simulink model "SIMULINK_FT_SRL_NZS_Tracking_R18b"  (R2018b)
settings: Solver=FixedStepAuto  StartTime=0.0  StopTime=sim_end_time  FixedStep=fixed_step_size  RelTol=1e-3
InitFcn:
  | start_uav_car_10
values from neighbouring files (symbols this model uses):
  a = 1    [start_uav_car_10.m]
  act_end = 2*pi/w1    (= 62.8318530718)    [start_uav_car_10.m]
  b = 1.8    [start_uav_car_10.m]
  battery_threshold = 20    [start_uav_car_10.m]
  bb = 1.2    [start_uav_car_10.m]
  delta_ = [delta_his(2:end,:); delta]    [adp_tracking.m]    (also in start_uav_car_10.m = zeros(N,1))
  draw_gif = false    [start_uav_car_10.m]
  fixed_step_size = 1/30    (= 0.0333333333333)    [start_uav_car_10.m]
  k = 0.2    [start_uav_car_10.m]
  KD_x = 0.000002    (= 2e-06)    [start_uav_car_10.m]
  KD_y = 0.00002    (= 2e-05)    [start_uav_car_10.m]
  kd_z = 0.02    [start_uav_car_10.m]
  KDD_x = 0.0008    [start_uav_car_10.m]
  KDD_y = 0.0008    [start_uav_car_10.m]
  KI_x = 0.000002    (= 2e-06)    [start_uav_car_10.m]
  KI_y = 0.000002    (= 2e-06)    [start_uav_car_10.m]
  ki_z = 0.002    [start_uav_car_10.m]
  KII_x = 0.000000    (= 0)    [start_uav_car_10.m]
  KII_y = 0.000    (= 0)    [start_uav_car_10.m]
  KP_x = 1.5    [start_uav_car_10.m]
  KP_y = 1.5    [start_uav_car_10.m]
  kp_z = 0.7    [start_uav_car_10.m]
  KPP_x = 0.4    [start_uav_car_10.m]
  KPP_y = 0.4    [start_uav_car_10.m]
  lmt = 0.5    [start_uav_car_10.m]
  omega = omega_(i,:)    [adp_tracking.m]    (also in start_uav_car_10.m = 0.3)
  omega_ = [omega_his(2:end,:); omega']    [adp_tracking.m]    (also in start_uav_car_10.m = zeros(N,l))
  R = 200*eye(2)    [adp_tracking.m]    (also in start_uav_car_10.m = 0.7)
  sim_end_time = 300    [start_uav_car_10.m]    (also in trjcar.m = 600)
  UAV_NUM = 1    [start_uav_car_10.m]
  Vel_Switch_1 = 1    [start_uav_car_10.m]
  Vel_Switch_10 = 1    [start_uav_car_10.m]
  Vel_Switch_11 = 1    [start_uav_car_10.m]
  Vel_Switch_12 = 1    [start_uav_car_10.m]
  Vel_Switch_13 = 1    [start_uav_car_10.m]
  Vel_Switch_14 = 1    [start_uav_car_10.m]
  Vel_Switch_15 = 1    [start_uav_car_10.m]
  Vel_Switch_16 = 1    [start_uav_car_10.m]
  Vel_Switch_17 = 1    [start_uav_car_10.m]
  Vel_Switch_18 = 1    [start_uav_car_10.m]
  Vel_Switch_19 = 1    [start_uav_car_10.m]
  Vel_Switch_2 = 1    [start_uav_car_10.m]
  Vel_Switch_20 = 1    [start_uav_car_10.m]
  Vel_Switch_3 = 1    [start_uav_car_10.m]
  Vel_Switch_4 = 1    [start_uav_car_10.m]
  Vel_Switch_5 = 1    [start_uav_car_10.m]
  Vel_Switch_6 = 1    [start_uav_car_10.m]
  Vel_Switch_7 = 1    [start_uav_car_10.m]
  Vel_Switch_8 = 1    [start_uav_car_10.m]
  Vel_Switch_9 = 1    [start_uav_car_10.m]
  W0 = 10*ones(l,1)    [start_uav_car_10.m]
  w1 = 0.1    [start_uav_car_10.m]
  w2 = 30    [start_uav_car_10.m]
  XMAX = 2.8    [start_uav_car_10.m]
  XMIN = -2.8    [start_uav_car_10.m]
  YMAX = 2.2    [start_uav_car_10.m]
  YMIN = -2.2    [start_uav_car_10.m]
  ys = ys_learned - ys_learned(1,:)    [start_uav_car_10.m]
  ys_learned = [-20 -19.9842645881 -19.9722755737 -19.9635643089 -19.9577075469 -19.9543235714 -19.9530686431 -19.9536337356 -19.9557415391 -19.9591437091 -19.9636183405 -19.9689676484 ... (12618 elements, 6309x2)]    [DMP_ref.mat]
  z_d_for_land = 1    [start_uav_car_10.m]
  ZMAX = 2.0    (= 2)    [start_uav_car_10.m]
  ZMIN = 0.7    [start_uav_car_10.m]
undefined symbols (not defined in the file or in its folder): droneyeeUAV2_NUM, droneyeeUAV3_NUM, droneyeeUAV4_NUM, droneyeeUAV5_NUM, uav10num, uav1num, uav2num, uav3num, uav4num, uav5num, uav6num, uav7num, uav8num, uav9num
libraries: simulink x121, aerolibanimutils x1
(part 9 of 11)

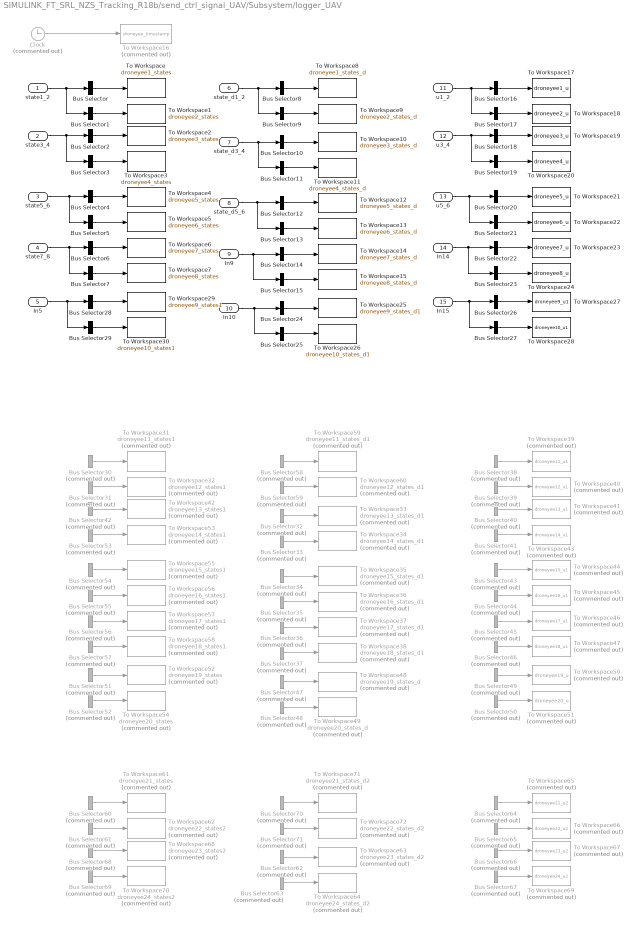
== system SIMULINK_FT_SRL_NZS_Tracking_R18b/send_ctrl_signal_UAV/Subsystem/logger_UAV ==
  state1_2 : Inport
  state3_4 : Inport  Port=2
  state5_6 : Inport  Port=3
  state7_8 : Inport  Port=4
  In5 : Inport  Port=5
  state_d1_2 : Inport  Port=6
  state_d3_4 : Inport  Port=7
  state_d5_6 : Inport  Port=8
  In9 : Inport  Port=9
  In10 : Inport  Port=10
  u1_2 : Inport  Port=11
  u3_4 : Inport  Port=12
  u5_6 : Inport  Port=13
  In14 : Inport  Port=14
  In15 : Inport  Port=15
  Bus Selector : BusSelector  OutputSignals=droneyeeUAV1_states.x,droneyeeUAV1_states.y,droneyeeUAV1_states.z,droneyeeUAV1_states.roll,droneyeeUAV1_states.pitch,droneyeeUAV1_states.yaw  OutputAsBus=on
  Bus Selector1 : BusSelector  OutputSignals=droneyeeUAV2_states.x,droneyeeUAV2_states.y,droneyeeUAV2_states.z,droneyeeUAV2_states.roll,droneyeeUAV2_states.pitch,droneyeeUAV2_states.yaw  OutputAsBus=on
  Bus Selector10 : BusSelector  OutputSignals=droneyeeUAV3_d.x3_d,droneyeeUAV3_d.y3_d,droneyeeUAV3_d.z3_d,droneyeeUAV3_d.yaw3_d  OutputAsBus=on
  Bus Selector11 : BusSelector  OutputSignals=droneyeeUAV4_d.x4_d,droneyeeUAV4_d.y4_d,droneyeeUAV4_d.z4_d,droneyeeUAV4_d.yaw4_d  OutputAsBus=on
  Bus Selector12 : BusSelector  OutputSignals=droneyeeUAV5_d.x5_d,droneyeeUAV5_d.y5_d,droneyeeUAV5_d.z5_d,droneyeeUAV5_d.yaw5_d  OutputAsBus=on
  Bus Selector13 : BusSelector  OutputSignals=droneyeeUAV6_d  OutputAsBus=on
  Bus Selector14 : BusSelector  OutputSignals=droneyeeUAV7_d  OutputAsBus=on
  Bus Selector15 : BusSelector  OutputSignals=droneyeeUAV8_d  OutputAsBus=on
  Bus Selector16 : BusSelector  OutputSignals=uav1.u_vx,uav1.u_vy,uav1.u_vz,uav1.u_rate_roll,uav1.u_rate_pitch,uav1.u_rate_yaw  OutputAsBus=on
  Bus Selector17 : BusSelector  OutputSignals=uav2.u_vx,uav2.u_vy,uav2.u_vz,uav2.u_rate_roll,uav2.u_rate_pitch,uav2.u_rate_yaw  OutputAsBus=on
  Bus Selector18 : BusSelector  OutputSignals=uav3.u_vx,uav3.u_vy,uav3.u_vz,uav3.u_rate_roll,uav3.u_rate_pitch,uav3.u_rate_yaw  OutputAsBus=on
  Bus Selector19 : BusSelector  OutputSignals=uav4.u_vx,uav4.u_vy,uav4.u_vz,uav4.u_rate_roll,uav4.u_rate_pitch,uav4.u_rate_yaw  OutputAsBus=on
  Bus Selector2 : BusSelector  OutputSignals=droneyeeUAV3_states.x,droneyeeUAV3_states.y,droneyeeUAV3_states.z,droneyeeUAV3_states.roll,droneyeeUAV3_states.pitch,droneyeeUAV3_states.yaw  OutputAsBus=on
  Bus Selector20 : BusSelector  OutputSignals=uav_5.u_vx,uav_5.u_vy,uav_5.u_vz,uav_5.u_rate_roll,uav_5.u_rate_pitch,uav_5.u_rate_yaw  OutputAsBus=on
  Bus Selector21 : BusSelector  OutputSignals=uav_6  OutputAsBus=on
  Bus Selector22 : BusSelector  OutputSignals=uav_7  OutputAsBus=on
  Bus Selector23 : BusSelector  OutputSignals=uav_8  OutputAsBus=on
  Bus Selector24 : BusSelector  OutputSignals=droneyeeUAV9_d  OutputAsBus=on
  Bus Selector25 : BusSelector  OutputSignals=droneyeeUAV10_d  OutputAsBus=on
  Bus Selector26 : BusSelector  OutputSignals=uav_9  OutputAsBus=on
  Bus Selector27 : BusSelector  OutputSignals=uav_10  OutputAsBus=on
  Bus Selector28 : BusSelector  OutputSignals=droneyeeUAV9_states  OutputAsBus=on
  Bus Selector29 : BusSelector  OutputSignals=droneyeeUAV10_states  OutputAsBus=on
  Bus Selector3 : BusSelector  OutputSignals=droneyeeUAV4_states.x,droneyeeUAV4_states.y,droneyeeUAV4_states.z,droneyeeUAV4_states.roll,droneyeeUAV4_states.pitch,droneyeeUAV4_states.yaw  OutputAsBus=on
  Bus Selector30 : BusSelector  Commented=on  OutputSignals=droneyeeUAV11_states.x1,droneyeeUAV11_states.y1,droneyeeUAV11_states.z1,droneyeeUAV11_states.yaw1,droneyeeUAV11_states.vx1,droneyeeUAV11_states.vy1,droneyeeUAV11_states.vz1  OutputAsBus=on
  Bus Selector31 : BusSelector  Commented=on  OutputSignals=droneyeeUAV12_states.x2,droneyeeUAV12_states.y2,droneyeeUAV12_states.z2,droneyeeUAV12_states.yaw2,droneyeeUAV12_states.vx2,droneyeeUAV12_states.vy2,droneyeeUAV12_states.vz2  OutputAsBus=on
  Bus Selector32 : BusSelector  Commented=on  OutputSignals=droneyeeUAV13_d.x13_d,droneyeeUAV13_d.y13_d,droneyeeUAV13_d.z13_d,droneyeeUAV13_d.yaw13_d  OutputAsBus=on
  Bus Selector33 : BusSelector  Commented=on  OutputSignals=droneyeeUAV14_d.x14_d,droneyeeUAV14_d.y14_d,droneyeeUAV14_d.z14_d,droneyeeUAV14_d.yaw14_d  OutputAsBus=on
  Bus Selector34 : BusSelector  Commented=on  OutputSignals=droneyeeUAV15_d.x15_d,droneyeeUAV15_d.y15_d,droneyeeUAV15_d.z15_d,droneyeeUAV15_d.yaw15_d  OutputAsBus=on
  Bus Selector35 : BusSelector  Commented=on  OutputSignals=droneyeeUAV16_d.x16_d,droneyeeUAV16_d.y16_d,droneyeeUAV16_d.z16_d,droneyeeUAV16_d.yaw16_d  OutputAsBus=on
  Bus Selector36 : BusSelector  Commented=on  OutputSignals=droneyeeUAV17_d.x17_d,droneyeeUAV17_d.y17_d,droneyeeUAV17_d.z17_d,droneyeeUAV17_d.yaw17_d  OutputAsBus=on
  Bus Selector37 : BusSelector  Commented=on  OutputSignals=droneyeeUAV18_d.x18_d,droneyeeUAV18_d.y18_d,droneyeeUAV18_d.z18_d,droneyeeUAV18_d.yaw18_d  OutputAsBus=on
  Bus Selector38 : BusSelector  Commented=on  OutputSignals=uav1.u_vx,uav1.u_vy,uav1.u_vz,uav1.u_rate_roll,uav1.u_rate_pitch,uav1.u_rate_yaw  OutputAsBus=on
  Bus Selector39 : BusSelector  Commented=on  OutputSignals=uav2.u_vx,uav2.u_vy,uav2.u_vz,uav2.u_rate_roll,uav2.u_rate_pitch,uav2.u_rate_yaw  OutputAsBus=on
  Bus Selector4 : BusSelector  OutputSignals=droneyeeUAV5_states.x,droneyeeUAV5_states.y,droneyeeUAV5_states.z,droneyeeUAV5_states.roll,droneyeeUAV5_states.pitch,droneyeeUAV5_states.yaw  OutputAsBus=on
  Bus Selector40 : BusSelector  Commented=on  OutputSignals=uav3.u_vx,uav3.u_vy,uav3.u_vz,uav3.u_rate_roll,uav3.u_rate_pitch,uav3.u_rate_yaw  OutputAsBus=on
  Bus Selector41 : BusSelector  Commented=on  OutputSignals=uav4.u_vx,uav4.u_vy,uav4.u_vz,uav4.u_rate_roll,uav4.u_rate_pitch,uav4.u_rate_yaw  OutputAsBus=on
  Bus Selector42 : BusSelector  Commented=on  OutputSignals=droneyeeUAV13_states.x3,droneyeeUAV13_states.y3,droneyeeUAV13_states.z3,droneyeeUAV13_states.yaw3,droneyeeUAV13_states.vx3,droneyeeUAV13_states.vy3,droneyeeUAV13_states.vz3  OutputAsBus=on
  Bus Selector43 : BusSelector  Commented=on  OutputSignals=uav5.u_vx,uav5.u_vy,uav5.u_vz,uav5.u_rate_roll,uav5.u_rate_pitch,uav5.u_rate_yaw  OutputAsBus=on
  Bus Selector44 : BusSelector  Commented=on  OutputSignals=uav6.u_vx,uav6.u_vy,uav6.u_vz,uav6.u_rate_roll,uav6.u_rate_pitch,uav6.u_rate_yaw  OutputAsBus=on
  Bus Selector45 : BusSelector  Commented=on  OutputSignals=uav7.u_vx,uav7.u_vy,uav7.u_vz,uav7.u_rate_roll,uav7.u_rate_pitch,uav7.u_rate_yaw  OutputAsBus=on
  Bus Selector46 : BusSelector  Commented=on  OutputSignals=uav8.u_vx,uav8.u_vy,uav8.u_vz,uav8.u_rate_roll,uav8.u_rate_pitch,uav8.u_rate_yaw  OutputAsBus=on
  Bus Selector47 : BusSelector  Commented=on  OutputSignals=droneyeeUAV19_d.x19_d,droneyeeUAV19_d.y19_d,droneyeeUAV19_d.z19_d,droneyeeUAV19_d.yaw19_d  OutputAsBus=on
  Bus Selector48 : BusSelector  Commented=on  OutputSignals=droneyeeUAV20_d.x20_d,droneyeeUAV20_d.y20_d,droneyeeUAV20_d.z20_d,droneyeeUAV20_d.yaw20_d  OutputAsBus=on
  Bus Selector49 : BusSelector  Commented=on  OutputSignals=uav9.u_vx,uav9.u_vy,uav9.u_vz,uav9.u_rate_roll,uav9.u_rate_pitch,uav9.u_rate_yaw  OutputAsBus=on
  Bus Selector5 : BusSelector  OutputSignals="droneyeeUAV6_states.x,droneyeeUAV6_states.y,droneyeeUAV6_states.z,droneyeeUAV6_states.roll,droneyeeUAV6_states.pitch,droneyeeUAV6_states.yaw,droneyeeUAV6_states.latitude(degE7),droneyeeUAV6_states.longitude\t(degE7),droneyeeUAV6_states.alttude(mm),droneyeeUAV6_states.x(home position),droneyeeUAV6_states.y(home position),droneyeeUAV6_states.z(home position)"  OutputAsBus=on
  Bus Selector50 : BusSelector  Commented=on  OutputSignals=uav10.u_vx,uav10.u_vy,uav10.u_vz,uav10.u_rate_roll,uav10.u_rate_pitch,uav10.u_rate_yaw  OutputAsBus=on
  Bus Selector51 : BusSelector  Commented=on  OutputSignals=droneyeeUAV19_states.x9,droneyeeUAV19_states.y9,droneyeeUAV19_states.z9,droneyeeUAV19_states.yaw9,droneyeeUAV19_states.vx9,droneyeeUAV19_states.vy9,droneyeeUAV19_states.vz9  OutputAsBus=on
  Bus Selector52 : BusSelector  Commented=on  OutputSignals=droneyeeUAV20_states.x10,droneyeeUAV20_states.y10,droneyeeUAV20_states.z10,droneyeeUAV20_states.yaw10,droneyeeUAV20_states.vx10,droneyeeUAV20_states.vy10,droneyeeUAV20_states.vz10  OutputAsBus=on
  Bus Selector53 : BusSelector  Commented=on  OutputSignals=droneyeeUAV14_states.x4,droneyeeUAV14_states.y4,droneyeeUAV14_states.z4,droneyeeUAV14_states.yaw4,droneyeeUAV14_states.vx4,droneyeeUAV14_states.vy4,droneyeeUAV14_states.vz4  OutputAsBus=on
  Bus Selector54 : BusSelector  Commented=on  OutputSignals=droneyeeUAV15_states.x5,droneyeeUAV15_states.y5,droneyeeUAV15_states.z5,droneyeeUAV15_states.yaw5,droneyeeUAV15_states.vx5,droneyeeUAV15_states.vy5,droneyeeUAV15_states.vz5  OutputAsBus=on
  Bus Selector55 : BusSelector  Commented=on  OutputSignals=droneyeeUAV16_states.x6,droneyeeUAV16_states.y6,droneyeeUAV16_states.z6,droneyeeUAV16_states.yaw6,droneyeeUAV16_states.vx6,droneyeeUAV16_states.vy6,droneyeeUAV16_states.vz6  OutputAsBus=on
  Bus Selector56 : BusSelector  Commented=on  OutputSignals=droneyeeUAV17_states.x7,droneyeeUAV17_states.y7,droneyeeUAV17_states.z7,droneyeeUAV17_states.yaw7,droneyeeUAV17_states.vx7,droneyeeUAV17_states.vy7,droneyeeUAV17_states.vz7  OutputAsBus=on
  Bus Selector57 : BusSelector  Commented=on  OutputSignals=droneyeeUAV18_states.x8,droneyeeUAV18_states.y8,droneyeeUAV18_states.z8,droneyeeUAV18_states.yaw8,droneyeeUAV18_states.vx8,droneyeeUAV18_states.vy8,droneyeeUAV18_states.vz8  OutputAsBus=on
  Bus Selector58 : BusSelector  Commented=on  OutputSignals=droneyeeUAV11_d.x11_d,droneyeeUAV11_d.y11_d,droneyeeUAV11_d.z11_d,droneyeeUAV11_d.yaw11_d  OutputAsBus=on
  Bus Selector59 : BusSelector  Commented=on  OutputSignals=droneyeeUAV12_d.x12_d,droneyeeUAV12_d.y12_d,droneyeeUAV12_d.z12_d,droneyeeUAV12_d.yaw12_d  OutputAsBus=on
  Bus Selector6 : BusSelector  OutputSignals=droneyeeUAV7_states  OutputAsBus=on
  Bus Selector60 : BusSelector  Commented=on  OutputSignals=droneyeeUAV21_states.x1,droneyeeUAV21_states.y1,droneyeeUAV21_states.z1,droneyeeUAV21_states.yaw1,droneyeeUAV21_states.vx1,droneyeeUAV21_states.vy1,droneyeeUAV21_states.vz1  OutputAsBus=on
  Bus Selector61 : BusSelector  Commented=on  OutputSignals=droneyeeUAV22_states.x2,droneyeeUAV22_states.y2,droneyeeUAV22_states.z2,droneyeeUAV22_states.yaw2,droneyeeUAV22_states.vx2,droneyeeUAV22_states.vy2,droneyeeUAV22_states.vz2  OutputAsBus=on
  Bus Selector62 : BusSelector  Commented=on  OutputSignals=droneyeeUAV23_d.x23_d,droneyeeUAV23_d.y23_d,droneyeeUAV23_d.z23_d,droneyeeUAV23_d.yaw23_d  OutputAsBus=on
  Bus Selector63 : BusSelector  Commented=on  OutputSignals=droneyeeUAV24_d.x24_d,droneyeeUAV24_d.y24_d,droneyeeUAV24_d.z24_d,droneyeeUAV24_d.yaw24_d  OutputAsBus=on
  Bus Selector64 : BusSelector  Commented=on  OutputSignals=uav1.u_vx,uav1.u_vy,uav1.u_vz,uav1.u_rate_roll,uav1.u_rate_pitch,uav1.u_rate_yaw  OutputAsBus=on
  Bus Selector65 : BusSelector  Commented=on  OutputSignals=uav2.u_vx,uav2.u_vy,uav2.u_vz,uav2.u_rate_roll,uav2.u_rate_pitch,uav2.u_rate_yaw  OutputAsBus=on
  Bus Selector66 : BusSelector  Commented=on  OutputSignals=uav3.u_vx,uav3.u_vy,uav3.u_vz,uav3.u_rate_roll,uav3.u_rate_pitch,uav3.u_rate_yaw  OutputAsBus=on
  Bus Selector67 : BusSelector  Commented=on  OutputSignals=uav4.u_vx,uav4.u_vy,uav4.u_vz,uav4.u_rate_roll,uav4.u_rate_pitch,uav4.u_rate_yaw  OutputAsBus=on
  Bus Selector68 : BusSelector  Commented=on  OutputSignals=droneyeeUAV23_states.x3,droneyeeUAV23_states.y3,droneyeeUAV23_states.z3,droneyeeUAV23_states.yaw3,droneyeeUAV23_states.vx3,droneyeeUAV23_states.vy3,droneyeeUAV23_states.vz3  OutputAsBus=on
  Bus Selector69 : BusSelector  Commented=on  OutputSignals=droneyeeUAV24_states.x4,droneyeeUAV24_states.y4,droneyeeUAV24_states.z4,droneyeeUAV24_states.yaw4,droneyeeUAV24_states.vx4,droneyeeUAV24_states.vy4,droneyeeUAV24_states.vz4  OutputAsBus=on
  Bus Selector7 : BusSelector  OutputSignals=droneyeeUAV8_states  OutputAsBus=on
  Bus Selector70 : BusSelector  Commented=on  OutputSignals=droneyeeUAV21_d.x21_d,droneyeeUAV21_d.y21_d,droneyeeUAV21_d.z21_d,droneyeeUAV21_d.yaw21_d  OutputAsBus=on
  Bus Selector71 : BusSelector  Commented=on  OutputSignals=droneyeeUAV22_d.x22_d,droneyeeUAV22_d.y22_d,droneyeeUAV22_d.z22_d,droneyeeUAV22_d.yaw22_d  OutputAsBus=on
  Bus Selector8 : BusSelector  OutputSignals=droneyeeUAV1_d.x1_d,droneyeeUAV1_d.y1_d,droneyeeUAV1_d.z1_d,droneyeeUAV1_d.yaw1_d  OutputAsBus=on
  Bus Selector9 : BusSelector  OutputSignals=droneyeeUAV2_d.x2_d,droneyeeUAV2_d.y2_d,droneyeeUAV2_d.z2_d,droneyeeUAV2_d.yaw2_d  OutputAsBus=on
  Clock : Clock  Commented=on
  To Workspace : ToWorkspace  VariableName=droneyee1_states  SampleTime=-1
  To Workspace1 : ToWorkspace  VariableName=droneyee2_states  SampleTime=-1
  To Workspace10 : ToWorkspace  VariableName=droneyee3_states_d  SampleTime=-1
  To Workspace11 : ToWorkspace  VariableName=droneyee4_states_d  SampleTime=-1
  To Workspace12 : ToWorkspace  VariableName=droneyee5_states_d  SampleTime=-1
  To Workspace13 : ToWorkspace  VariableName=droneyee6_states_d  SampleTime=-1
  To Workspace14 : ToWorkspace  VariableName=droneyee7_states_d  SampleTime=-1
  To Workspace15 : ToWorkspace  VariableName=droneyee8_states_d  SampleTime=-1
  To Workspace16 : ToWorkspace  Commented=on  VariableName=droneyee_timestamp  SampleTime=-1
  To Workspace17 : ToWorkspace  VariableName=droneyee1_u  SampleTime=-1
  To Workspace18 : ToWorkspace  VariableName=droneyee2_u  SampleTime=-1
  To Workspace19 : ToWorkspace  VariableName=droneyee3_u  SampleTime=-1
  To Workspace2 : ToWorkspace  VariableName=droneyee3_states  SampleTime=-1
  To Workspace20 : ToWorkspace  VariableName=droneyee4_u  SampleTime=-1
  To Workspace21 : ToWorkspace  VariableName=droneyee5_u  SampleTime=-1
  To Workspace22 : ToWorkspace  VariableName=droneyee6_u  SampleTime=-1
  To Workspace23 : ToWorkspace  VariableName=droneyee7_u  SampleTime=-1
  To Workspace24 : ToWorkspace  VariableName=droneyee8_u  SampleTime=-1
  To Workspace25 : ToWorkspace  VariableName=droneyee9_states_d1  SampleTime=-1
  To Workspace26 : ToWorkspace  VariableName=droneyee10_states_d1  SampleTime=-1
  To Workspace27 : ToWorkspace  VariableName=droneyee9_u1  SampleTime=-1
  To Workspace28 : ToWorkspace  VariableName=droneyee10_u1  SampleTime=-1
  To Workspace29 : ToWorkspace  VariableName=droneyee9_states1  SampleTime=-1
  To Workspace3 : ToWorkspace  VariableName=droneyee4_states  SampleTime=-1
  To Workspace30 : ToWorkspace  VariableName=droneyee10_states1  SampleTime=-1
  To Workspace31 : ToWorkspace  Commented=on  VariableName=droneyee11_states1  SampleTime=-1
  To Workspace32 : ToWorkspace  Commented=on  VariableName=droneyee12_states1  SampleTime=-1
  To Workspace33 : ToWorkspace  Commented=on  VariableName=droneyee13_states_d1  SampleTime=-1
  To Workspace34 : ToWorkspace  Commented=on  VariableName=droneyee14_states_d1  SampleTime=-1
  To Workspace35 : ToWorkspace  Commented=on  VariableName=droneyee15_states_d1  SampleTime=-1
  To Workspace36 : ToWorkspace  Commented=on  VariableName=droneyee16_states_d1  SampleTime=-1
  To Workspace37 : ToWorkspace  Commented=on  VariableName=droneyee17_states_d1  SampleTime=-1
  To Workspace38 : ToWorkspace  Commented=on  VariableName=droneyee18_states_d1  SampleTime=-1
  To Workspace39 : ToWorkspace  Commented=on  VariableName=droneyee11_u1  SampleTime=-1
  To Workspace4 : ToWorkspace  VariableName=droneyee5_states  SampleTime=-1
  To Workspace40 : ToWorkspace  Commented=on  VariableName=droneyee12_u1  SampleTime=-1
  To Workspace41 : ToWorkspace  Commented=on  VariableName=droneyee13_u1  SampleTime=-1
  To Workspace42 : ToWorkspace  Commented=on  VariableName=droneyee13_states1  SampleTime=-1
  To Workspace43 : ToWorkspace  Commented=on  VariableName=droneyee14_u1  SampleTime=-1
  To Workspace44 : ToWorkspace  Commented=on  VariableName=droneyee15_u1  SampleTime=-1
  To Workspace45 : ToWorkspace  Commented=on  VariableName=droneyee16_u1  SampleTime=-1
  To Workspace46 : ToWorkspace  Commented=on  VariableName=droneyee17_u1  SampleTime=-1
  To Workspace47 : ToWorkspace  Commented=on  VariableName=droneyee18_u1  SampleTime=-1
  To Workspace48 : ToWorkspace  Commented=on  VariableName=droneyee19_states_d  SampleTime=-1
  To Workspace49 : ToWorkspace  Commented=on  VariableName=droneyee20_states_d  SampleTime=-1
  To Workspace5 : ToWorkspace  VariableName=droneyee6_states  SampleTime=-1
  To Workspace50 : ToWorkspace  Commented=on  VariableName=droneyee19_u  SampleTime=-1
  To Workspace51 : ToWorkspace  Commented=on  VariableName=droneyee20_u  SampleTime=-1
  To Workspace52 : ToWorkspace  Commented=on  VariableName=droneyee19_states  SampleTime=-1
  To Workspace53 : ToWorkspace  Commented=on  VariableName=droneyee14_states1  SampleTime=-1
  To Workspace54 : ToWorkspace  Commented=on  VariableName=droneyee20_states  SampleTime=-1
  To Workspace55 : ToWorkspace  Commented=on  VariableName=droneyee15_states1  SampleTime=-1
  To Workspace56 : ToWorkspace  Commented=on  VariableName=droneyee16_states1  SampleTime=-1
  To Workspace57 : ToWorkspace  Commented=on  VariableName=droneyee17_states1  SampleTime=-1
  To Workspace58 : ToWorkspace  Commented=on  VariableName=droneyee18_states1  SampleTime=-1
  To Workspace59 : ToWorkspace  Commented=on  VariableName=droneyee11_states_d1  SampleTime=-1
  To Workspace6 : ToWorkspace  VariableName=droneyee7_states  SampleTime=-1
  To Workspace60 : ToWorkspace  Commented=on  VariableName=droneyee12_states_d1  SampleTime=-1
  To Workspace61 : ToWorkspace  Commented=on  VariableName=droneyee21_states  SampleTime=-1
  To Workspace62 : ToWorkspace  Commented=on  VariableName=droneyee22_states2  SampleTime=-1
  To Workspace63 : ToWorkspace  Commented=on  VariableName=droneyee23_states_d2  SampleTime=-1
  To Workspace64 : ToWorkspace  Commented=on  VariableName=droneyee24_states_d2  SampleTime=-1
  To Workspace65 : ToWorkspace  Commented=on  VariableName=droneyee21_u2  SampleTime=-1
  To Workspace66 : ToWorkspace  Commented=on  VariableName=droneyee22_u2  SampleTime=-1
  To Workspace67 : ToWorkspace  Commented=on  VariableName=droneyee23_u2  SampleTime=-1
  To Workspace68 : ToWorkspace  Commented=on  VariableName=droneyee23_states2  SampleTime=-1
  To Workspace69 : ToWorkspace  Commented=on  VariableName=droneyee24_u2  SampleTime=-1
  To Workspace7 : ToWorkspace  VariableName=droneyee8_states  SampleTime=-1
  To Workspace70 : ToWorkspace  Commented=on  VariableName=droneyee24_states2  SampleTime=-1
  To Workspace71 : ToWorkspace  Commented=on  VariableName=droneyee21_states_d2  SampleTime=-1
  To Workspace72 : ToWorkspace  Commented=on  VariableName=droneyee22_states_d2  SampleTime=-1
  To Workspace8 : ToWorkspace  VariableName=droneyee1_states_d  SampleTime=-1
  To Workspace9 : ToWorkspace  VariableName=droneyee2_states_d  SampleTime=-1
  wires:
  state1_2/1 -> Bus Selector1/1, Bus Selector/1
  Bus Selector/1 -> To Workspace/1
  Bus Selector1/1 -> To Workspace1/1
  Bus Selector3/1 -> To Workspace3/1
  Bus Selector2/1 -> To Workspace2/1
  state3_4/1 -> Bus Selector3/1, Bus Selector2/1
  Bus Selector5/1 -> To Workspace5/1
  Bus Selector4/1 -> To Workspace4/1
  Bus Selector7/1 -> To Workspace7/1
  Bus Selector6/1 -> To Workspace6/1
  Bus Selector9/1 -> To Workspace9/1
  Bus Selector8/1 -> To Workspace8/1
  state_d1_2/1 -> Bus Selector9/1, Bus Selector8/1
  Bus Selector10/1 -> To Workspace10/1
  Bus Selector11/1 -> To Workspace11/1
  Bus Selector12/1 -> To Workspace12/1
  state_d3_4/1 -> Bus Selector11/1, Bus Selector10/1
  state_d5_6/1 -> Bus Selector13/1, Bus Selector12/1
  Bus Selector15/1 -> To Workspace15/1
  Bus Selector13/1 -> To Workspace13/1
  Bus Selector14/1 -> To Workspace14/1
  Clock/1 -> To Workspace16/1
  Bus Selector18/1 -> To Workspace19/1
  Bus Selector19/1 -> To Workspace20/1
  Bus Selector20/1 -> To Workspace21/1
  u5_6/1 -> Bus Selector21/1, Bus Selector20/1
  Bus Selector21/1 -> To Workspace22/1
  Bus Selector23/1 -> To Workspace24/1
  u1_2/1 -> Bus Selector17/1, Bus Selector16/1
  Bus Selector17/1 -> To Workspace18/1
  Bus Selector16/1 -> To Workspace17/1
  u3_4/1 -> Bus Selector19/1, Bus Selector18/1
  Bus Selector22/1 -> To Workspace23/1
  Bus Selector27/1 -> To Workspace28/1
  Bus Selector26/1 -> To Workspace27/1
  Bus Selector29/1 -> To Workspace30/1
  Bus Selector25/1 -> To Workspace26/1
  Bus Selector28/1 -> To Workspace29/1
  Bus Selector24/1 -> To Workspace25/1
  Bus Selector40/1 -> To Workspace41/1
  Bus Selector36/1 -> To Workspace37/1
  Bus Selector55/1 -> To Workspace56/1
  Bus Selector43/1 -> To Workspace44/1
  Bus Selector48/1 -> To Workspace49/1
  Bus Selector52/1 -> To Workspace54/1
  Bus Selector34/1 -> To Workspace35/1
  Bus Selector39/1 -> To Workspace40/1
  Bus Selector35/1 -> To Workspace36/1
  Bus Selector47/1 -> To Workspace48/1
  Bus Selector54/1 -> To Workspace55/1
  Bus Selector37/1 -> To Workspace38/1
  Bus Selector42/1 -> To Workspace42/1
  Bus Selector56/1 -> To Workspace57/1
  Bus Selector58/1 -> To Workspace59/1
  Bus Selector32/1 -> To Workspace33/1
  Bus Selector57/1 -> To Workspace58/1
  Bus Selector30/1 -> To Workspace31/1
  Bus Selector45/1 -> To Workspace46/1
  Bus Selector31/1 -> To Workspace32/1
  Bus Selector33/1 -> To Workspace34/1
  Bus Selector59/1 -> To Workspace60/1
  Bus Selector44/1 -> To Workspace45/1
  Bus Selector46/1 -> To Workspace47/1
  Bus Selector51/1 -> To Workspace52/1
  Bus Selector53/1 -> To Workspace53/1
  Bus Selector38/1 -> To Workspace39/1
  Bus Selector50/1 -> To Workspace51/1
  Bus Selector49/1 -> To Workspace50/1
  Bus Selector41/1 -> To Workspace43/1
  Bus Selector68/1 -> To Workspace68/1
  Bus Selector67/1 -> To Workspace69/1
  Bus Selector69/1 -> To Workspace70/1
  Bus Selector71/1 -> To Workspace72/1
  Bus Selector66/1 -> To Workspace67/1
  Bus Selector62/1 -> To Workspace63/1
  Bus Selector61/1 -> To Workspace62/1
  Bus Selector63/1 -> To Workspace64/1
  Bus Selector65/1 -> To Workspace66/1
  Bus Selector60/1 -> To Workspace61/1
  Bus Selector64/1 -> To Workspace65/1
  Bus Selector70/1 -> To Workspace71/1
  state7_8/1 -> Bus Selector7/1, Bus Selector6/1
  state5_6/1 -> Bus Selector5/1, Bus Selector4/1
  In9/1 -> Bus Selector15/1, Bus Selector14/1
  In5/1 -> Bus Selector29/1, Bus Selector28/1
  In10/1 -> Bus Selector25/1, Bus Selector24/1
  In14/1 -> Bus Selector23/1, Bus Selector22/1
  In15/1 -> Bus Selector27/1, Bus Selector26/1

== system SIMULINK_FT_SRL_NZS_Tracking_R18b/send_ctrl_signal_car1/Send Command 1/Subsystem ==
  In1 : Inport
  Compare To Constant2 : simulink/Logic and Bit Operations/Compare To Constant  relop=~=  const=0  OutDataTypeStr=boolean
  Demux : Demux  Outputs=2
  Logical Operator1 : Logic  Operator=OR  AllPortsSameDT=off  OutDataTypeStr=boolean
  Out1 : Outport
  wires:
  Demux/2 -> Logical Operator1/2
  Logical Operator1/1 -> Out1/1
  Demux/1 -> Logical Operator1/1
  Compare To Constant2/1 -> Demux/1
  In1/1 -> Compare To Constant2/1

== system SIMULINK_FT_SRL_NZS_Tracking_R18b/send_ctrl_signal_car1/Send Command 10/Subsystem ==
  In1 : Inport
  Compare To Constant2 : simulink/Logic and Bit Operations/Compare To Constant  relop=~=  const=0  OutDataTypeStr=boolean
  Demux : Demux  Outputs=2
  Logical Operator1 : Logic  Operator=OR  AllPortsSameDT=off  OutDataTypeStr=boolean
  Out1 : Outport
  wires:
  Demux/2 -> Logical Operator1/2
  Logical Operator1/1 -> Out1/1
  Demux/1 -> Logical Operator1/1
  Compare To Constant2/1 -> Demux/1
  In1/1 -> Compare To Constant2/1

== system SIMULINK_FT_SRL_NZS_Tracking_R18b/send_ctrl_signal_car1/Send Command 2/Subsystem ==
  In1 : Inport
  Compare To Constant2 : simulink/Logic and Bit Operations/Compare To Constant  relop=~=  const=0  OutDataTypeStr=boolean
  Demux : Demux  Outputs=2
  Logical Operator1 : Logic  Operator=OR  AllPortsSameDT=off  OutDataTypeStr=boolean
  Out1 : Outport
  wires:
  Demux/2 -> Logical Operator1/2
  Logical Operator1/1 -> Out1/1
  Demux/1 -> Logical Operator1/1
  Compare To Constant2/1 -> Demux/1
  In1/1 -> Compare To Constant2/1

== system SIMULINK_FT_SRL_NZS_Tracking_R18b/send_ctrl_signal_car1/Send Command 3/Subsystem ==
  In1 : Inport
  Compare To Constant2 : simulink/Logic and Bit Operations/Compare To Constant  relop=~=  const=0  OutDataTypeStr=boolean
  Demux : Demux  Outputs=2
  Logical Operator1 : Logic  Operator=OR  AllPortsSameDT=off  OutDataTypeStr=boolean
  Out1 : Outport
  wires:
  Demux/2 -> Logical Operator1/2
  Logical Operator1/1 -> Out1/1
  Demux/1 -> Logical Operator1/1
  Compare To Constant2/1 -> Demux/1
  In1/1 -> Compare To Constant2/1

== system SIMULINK_FT_SRL_NZS_Tracking_R18b/send_ctrl_signal_car1/Send Command 4/Subsystem ==
  In1 : Inport
  Compare To Constant2 : simulink/Logic and Bit Operations/Compare To Constant  relop=~=  const=0  OutDataTypeStr=boolean
  Demux : Demux  Outputs=2
  Logical Operator1 : Logic  Operator=OR  AllPortsSameDT=off  OutDataTypeStr=boolean
  Out1 : Outport
  wires:
  Demux/2 -> Logical Operator1/2
  Logical Operator1/1 -> Out1/1
  Demux/1 -> Logical Operator1/1
  Compare To Constant2/1 -> Demux/1
  In1/1 -> Compare To Constant2/1

== system SIMULINK_FT_SRL_NZS_Tracking_R18b/send_ctrl_signal_car1/Send Command 5/Subsystem ==
  In1 : Inport
  Compare To Constant2 : simulink/Logic and Bit Operations/Compare To Constant  relop=~=  const=0  OutDataTypeStr=boolean
  Demux : Demux  Outputs=2
  Logical Operator1 : Logic  Operator=OR  AllPortsSameDT=off  OutDataTypeStr=boolean
  Out1 : Outport
  wires:
  Demux/2 -> Logical Operator1/2
  Logical Operator1/1 -> Out1/1
  Demux/1 -> Logical Operator1/1
  Compare To Constant2/1 -> Demux/1
  In1/1 -> Compare To Constant2/1

== system SIMULINK_FT_SRL_NZS_Tracking_R18b/send_ctrl_signal_car1/Send Command 6/Subsystem ==
  In1 : Inport
  Compare To Constant2 : simulink/Logic and Bit Operations/Compare To Constant  relop=~=  const=0  OutDataTypeStr=boolean
  Demux : Demux  Outputs=2
  Logical Operator1 : Logic  Operator=OR  AllPortsSameDT=off  OutDataTypeStr=boolean
  Out1 : Outport
  wires:
  Demux/2 -> Logical Operator1/2
  Logical Operator1/1 -> Out1/1
  Demux/1 -> Logical Operator1/1
  Compare To Constant2/1 -> Demux/1
  In1/1 -> Compare To Constant2/1

== system SIMULINK_FT_SRL_NZS_Tracking_R18b/send_ctrl_signal_car1/Send Command 7/Subsystem ==
  In1 : Inport
  Compare To Constant2 : simulink/Logic and Bit Operations/Compare To Constant  relop=~=  const=0  OutDataTypeStr=boolean
  Demux : Demux  Outputs=2
  Logical Operator1 : Logic  Operator=OR  AllPortsSameDT=off  OutDataTypeStr=boolean
  Out1 : Outport
  wires:
  Demux/2 -> Logical Operator1/2
  Logical Operator1/1 -> Out1/1
  Demux/1 -> Logical Operator1/1
  Compare To Constant2/1 -> Demux/1
  In1/1 -> Compare To Constant2/1

== system SIMULINK_FT_SRL_NZS_Tracking_R18b/send_ctrl_signal_car1/Send Command 8/Subsystem ==
  In1 : Inport
  Compare To Constant2 : simulink/Logic and Bit Operations/Compare To Constant  relop=~=  const=0  OutDataTypeStr=boolean
  Demux : Demux  Outputs=2
  Logical Operator1 : Logic  Operator=OR  AllPortsSameDT=off  OutDataTypeStr=boolean
  Out1 : Outport
  wires:
  Demux/2 -> Logical Operator1/2
  Logical Operator1/1 -> Out1/1
  Demux/1 -> Logical Operator1/1
  Compare To Constant2/1 -> Demux/1
  In1/1 -> Compare To Constant2/1

== system SIMULINK_FT_SRL_NZS_Tracking_R18b/send_ctrl_signal_car1/Send Command 9/Subsystem ==
  In1 : Inport
  Compare To Constant2 : simulink/Logic and Bit Operations/Compare To Constant  relop=~=  const=0  OutDataTypeStr=boolean
  Demux : Demux  Outputs=2
  Logical Operator1 : Logic  Operator=OR  AllPortsSameDT=off  OutDataTypeStr=boolean
  Out1 : Outport
  wires:
  Demux/2 -> Logical Operator1/2
  Logical Operator1/1 -> Out1/1
  Demux/1 -> Logical Operator1/1
  Compare To Constant2/1 -> Demux/1
  In1/1 -> Compare To Constant2/1
